simulink model "oTTo_Model2"  (R2021a)
settings: Solver=VariableStepAuto  StartTime=0.0  StopTime=inf  RelTol=1e-3
libraries: simulink x1
settings Model: SimulationMode=accelerator  PacingRate=100  Creator=an107  LastModifiedBy=an107

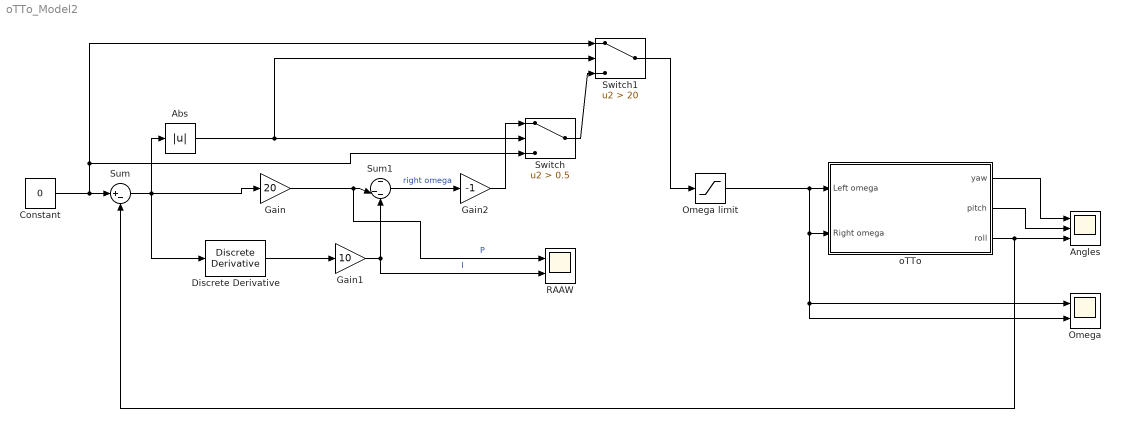
== system oTTo_Model2 ==
  Abs : Abs
  Angles : Scope  NumInputPorts=3
  Constant : Constant  Value=0
  Discrete Derivative : simulink/Discrete/Discrete Derivative  gainval=1.0  ICPrevScaledInput=0.0  OutMin=[]  OutMax=[]  OutDataType=fixdt(1, 16)  OutScaling=2^-10  DoSatur=off
  Gain : Gain  Gain=20
  Gain1 : Gain  Gain=10
  Gain2 : Gain  Gain=-1
  Omega : Scope  NumInputPorts=2
  Omega limit : Saturate  UpperLimit=720  LowerLimit=-720
  RAAW : Scope  NumInputPorts=2
  Sum : Sum  Inputs=|+-
  Sum1 : Sum  Inputs=-|--
  Switch : Switch  Criteria=u2 > Threshold  Threshold=0.5  SaturateOnIntegerOverflow=on
  Switch1 : Switch  Criteria=u2 > Threshold  Threshold=20  SaturateOnIntegerOverflow=on
  oTTo : Subsystem
  wires:
  oTTo/1(yaw) -> Angles/1
  oTTo/2(pitch) -> Angles/2
  oTTo/3(roll) -> Angles/3, Sum/2
  Constant/1 -> Switch1/1, Switch/3, Sum/1
  Gain/1 -> RAAW/1, Sum1/2  "P"
  Gain1/1 -> Sum1/3, RAAW/2  "I"
  Sum/1 -> Discrete Derivative/1, Abs/1, Gain/1
  Sum1/1 -> Gain2/1  "right omega"
  Omega limit/1 -> oTTo/1(Left omega), Omega/2, Omega/1, oTTo/2(Right omega)
  Abs/1 -> Switch1/2, Switch/2
  Gain2/1 -> Switch/1
  Discrete Derivative/1 -> Gain1/1
  Switch/1 -> Switch1/3
  Switch1/1 -> Omega limit/1

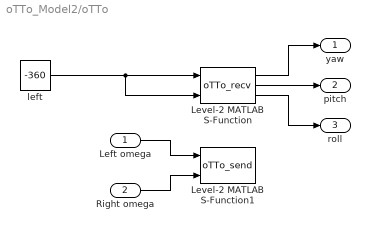
== system oTTo_Model2/oTTo ==
  Left omega : Inport
  Right omega : Inport  Port=2
  Level-2 MATLAB S-Function : M-S-Function  FunctionName=oTTo_recv  Parameters="\"COM4\", 115200,uart"
  Level-2 MATLAB S-Function1 : M-S-Function  FunctionName=oTTo_send  Parameters="\"COM4\", 115200,uart"
  left : Constant  Value=-360
  yaw : Outport
  pitch : Outport  Port=2
  roll : Outport  Port=3
  wires:
  left/1 -> Level-2 MATLAB S-Function/2, Level-2 MATLAB S-Function/1
  Left omega/1 -> Level-2 MATLAB S-Function1/1
  Right omega/1 -> Level-2 MATLAB S-Function1/2
  Level-2 MATLAB S-Function/1 -> yaw/1
  Level-2 MATLAB S-Function/2 -> pitch/1
  Level-2 MATLAB S-Function/3 -> roll/1
